simulink model "Practica_7simulink"  (R2024b)
settings: Solver=VariableStepAuto  StartTime=0.0  StopTime=10  RelTol=1e-3
InitFcn:
  | R1=5000000;
  | R2=5000000;
  | R3=5000000;
  | C1=.0000001;
  | C2=.0000001;
settings Model: Creator=Becho

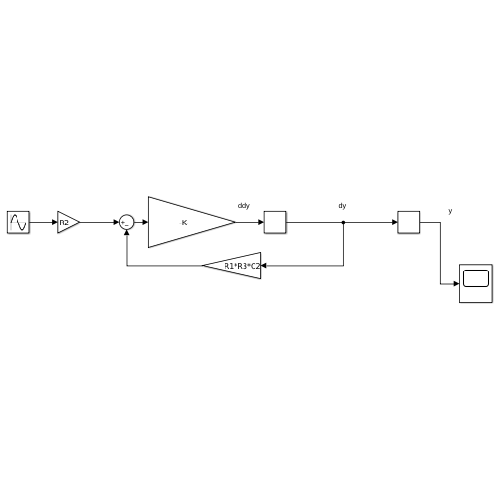
[thumbnail: Simulink's stored preview of the top-level diagram]
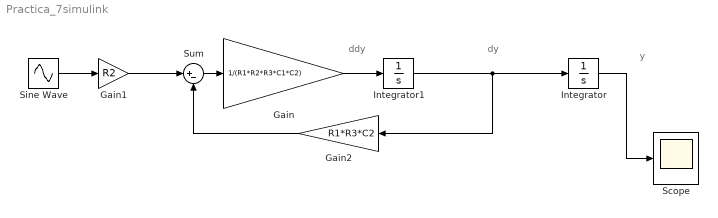
== system Practica_7simulink ==
  note: ddy
  note: dy
  note: y
  Gain : Gain  Gain=1/(R1*R2*R3*C1*C2)
  Gain1 : Gain  Gain=R2
  Gain2 : Gain  Gain=R1*R3*C2
  Integrator : Integrator
  Integrator1 : Integrator
  Scope : Scope
  Sine Wave : Sin  Frequency=628.32  SampleTime=0
  Sum : Sum  Inputs=|+-
  wires:
  Integrator1/1 -> Gain2/1, Integrator/1
  Gain/1 -> Integrator1/1
  Sum/1 -> Gain/1
  Sine Wave/1 -> Gain1/1
  Gain1/1 -> Sum/1
  Gain2/1 -> Sum/2
  Integrator/1 -> Scope/1
